simulink model "sltankrule"  (Simulink 4.00)
settings: Solver=ode45  SolverMode=SingleTasking  StartTime=0  StopTime=10000  MaxStep=0.2  RelTol=1e-3  AbsTol=1e-6
PreLoadFcn:
  | tank=readfis('tank');
libraries: fuzblock x1
CloseFcn:
  | AnimFigH = findobj(0,'Name', 'Tank Demo'); close(AnimFigH),ruleFigH = findobj(0,'Name', 'Rule Viewer: tank'); close(ruleFigH)
settings Model: Creator=pascal  LastModifiedBy=eyarrow  SaveTime=off  SaveOutput=off  LimitDataPoints=off  RTWTemplateMakefile=grt_unix.tmf  BlockReductionOpt=off

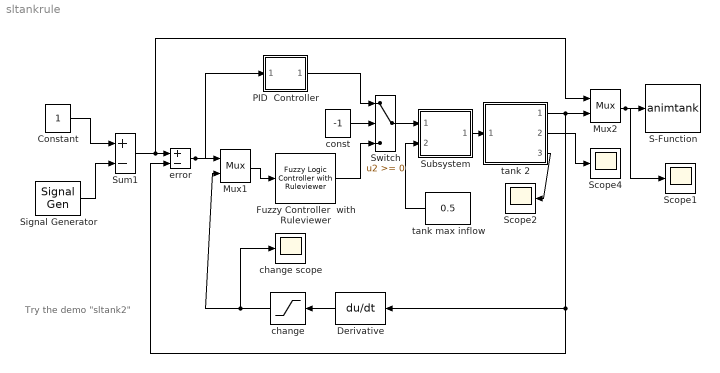
== system sltankrule ==
  note: Try the demo
      | "sltank2"
  Constant : Constant  Value=1
  Derivative : Derivative  Orientation=left
  Fuzzy Controller  with Ruleviewer : fuzblock/Fuzzy Logic  Controller  with Ruleviewer  fismatrix=tank  Ts=2
  Mux1 : Mux  Inputs=2
      settings: DisplayOption=none
  Mux2 : Mux  Inputs=2
      settings: DisplayOption=none
  PID  Controller : Subsystem  mask(PID Controller){@1=2, @2=0, @3=1}
      mask prompts: @1 "Proportional:"; @2 "Integral"; @3 "Derivative:"
      mask help:
      | Enter expressions for proportional, integral, and derivative terms.
      | P+I/s+Ds
      mask init:
      | P=@1; I=@2; D=@3;
      settings: RTWFcnNameOpts=Auto  RTWFileNameOpts=Auto
      mask Help: This block implements a PID controller where parameters are entered for the Proportional, Integral and Derivative terms. Unmask this block to see how it works. The derivative term is implemented using a true derivative block.
      mask Display: disp('PID')
  S-Function : S-Function  FunctionName=animtank  Parameters=1  PortCounts=[]  SFunctionModules=''
  Scope1 : Scope
      settings: TickLabels=on  TimeRange=200.000000  YMin=-2.000000  YMax=2.000000  SaveToWorkspace=off  SaveName=ScopeData  DataFormat=Array  LimitDataPoints=on  MaxDataPoints=5000
  Scope2 : Scope
      settings: TickLabels=on  TimeRange=20.000000  YMin=-2.000000  YMax=2.000000  SaveToWorkspace=off  SaveName=ScopeData  DataFormat=Array  LimitDataPoints=on  MaxDataPoints=5000
  Scope4 : Scope
      settings: TickLabels=on  TimeRange=200.000000  YMin=-2.000000  YMax=2.000000  SaveToWorkspace=off  SaveName=ScopeData  DataFormat=Array  LimitDataPoints=on  MaxDataPoints=5000
  Signal Generator : SignalGenerator  WaveForm=square  Amplitude=0.500000  Frequency=0.100000  Units=rad/sec
  Subsystem : Subsystem  mask(Valve){@1=0}
      mask prompts: @1 "Initial position [0=closed 1=open]:"
      mask help: Valve
      mask init:
      | InitialPosition = @1;
      settings: RTWFcnNameOpts=Auto  RTWFileNameOpts=Auto
      mask Display: disp('VALVE')
  Sum1 : Sum  Inputs=+-  SaturateOnIntegerOverflow=on
  Switch : Switch  Threshold=0
  change : Saturate  Orientation=left  UpperLimit=0.1  LowerLimit=-0.1  LinearizeAsGain=on
  change scope : Scope
      settings: TickLabels=on  TimeRange=20.000000  YMin=-0.100000  YMax=0.100000  SaveToWorkspace=off  SaveName=ScopeData  DataFormat=Array  LimitDataPoints=on  MaxDataPoints=5000
  const : Constant  Value=-1
  error : Sum  Inputs=+-  SaturateOnIntegerOverflow=on
  tank 2 : Subsystem  mask(Water tank){@1=2, @2=1, @3=0.05, @4=0, @5=0.5}
      mask prompts: @1 "Height of tank (m):"; @2 "Bottom area (m^2):"; @3 "Out pipe crossection (m^2):"; @4 "Overflow sensor distance from top (m):"; @5 "Initial level height (m):"
      mask help: Cylindrical water tank with overflow signal
      mask init:
      | ht=@1;area=@2;outletArea=@3;overflowLimit=@4;initialHt=@5;
      settings: RTWFcnNameOpts=Auto  RTWFileNameOpts=Auto
      mask Display: disp('WATER\nTANK')
  tank max inflow : Constant  Orientation=left  Value=0.5
  wires:
  tank 2/2(flow out) -> Scope4/1
  tank max inflow/1 -> Subsystem/2(source flow)
  Derivative/1 -> change/1
  Mux1/1 -> Fuzzy Controller  with Ruleviewer/1
  change/1 -> Mux1/2, change scope/1
  Constant/1 -> Sum1/1
  Signal Generator/1 -> Sum1/2
  Subsystem/1(out flow) -> tank 2/1(flow in)
  tank 2/1(water level) -> Mux2/2, error/2, Derivative/1
  Sum1/1 -> error/1, Mux2/1
  tank 2/3(overflow flag) -> Scope2/1
  Switch/1 -> Subsystem/1(control)
  Mux2/1 -> S-Function/1, Scope1/1
  error/1 -> Mux1/1, PID  Controller/1(In_1)
  Fuzzy Controller  with Ruleviewer/1 -> Switch/3
  PID  Controller/1(Out_1) -> Switch/1
  const/1 -> Switch/2

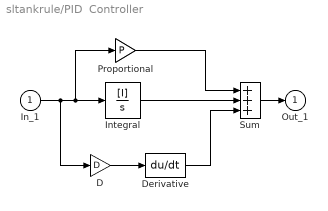
== system sltankrule/PID  Controller ==
  In_1 : Inport  Port=1  LatchInput=off
  D : Gain  Gain=D  Multiplication=Element-wise(K.*u)  SaturateOnIntegerOverflow=on
  Derivative : Derivative
  Integral : TransferFcn  Numerator=[I]  Denominator=[1 0]  AbsoluteTolerance=auto  Realization=auto
  Proportional : Gain  Gain=P  Multiplication=Element-wise(K.*u)  SaturateOnIntegerOverflow=on
  Sum : Sum  Inputs=+++  SaturateOnIntegerOverflow=on
  Out_1 : Outport  Port=1  InitialOutput=0
  wires:
  Proportional/1 -> Sum/1
  Integral/1 -> Sum/2
  Derivative/1 -> Sum/3
  In_1/1 -> Integral/1, Proportional/1, D/1
  Sum/1 -> Out_1/1
  D/1 -> Derivative/1

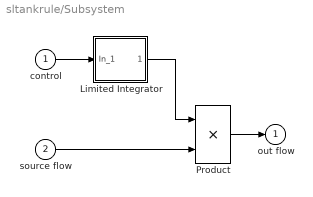
== system sltankrule/Subsystem ==
  control : Inport  Port=1  LatchInput=off
  source flow : Inport  Port=2  LatchInput=off
  Limited Integrator : Subsystem  mask(Limited integrator.){@1=0, @2=1, @3=InitialPosition}
      mask prompts: @1 "Lower bound:"; @2 "Upper bound:"; @3 "Initial condition"
      mask help: Limited integrator
      mask init:
      | lb = @1; ub = @2; xi = @3;
      settings: RTWFcnNameOpts=Auto  RTWFileNameOpts=Auto
      mask Help: Implements a limited integrator with \nan expression of the form:\n\nif(x<=lb and u<0) or (x>=ub and u>0)\n\txdot=0\nelse\n\txdot=u.
      mask Display: plot(-1,-0.2,3.5,1.2,[0.05,1,2,2.9],[0,0,1,1]);disp(' 1/s    ')
  Product : Product  Inputs=2  Multiplication=Element-wise(.*)  SaturateOnIntegerOverflow=on
  out flow : Outport  Port=1  InitialOutput=0
  wires:
  source flow/1 -> Product/2
  Product/1 -> out flow/1
  control/1 -> Limited Integrator/1(In_1)
  Limited Integrator/1(Out_1) -> Product/1

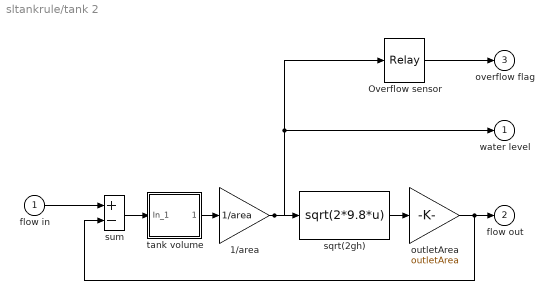
== system sltankrule/tank 2 ==
  flow in : Inport  Port=1  LatchInput=off
  1/area : Gain  Gain=1/area  Multiplication=Element-wise(K.*u)  SaturateOnIntegerOverflow=on
  Overflow sensor : Relay  OnSwitchValue=ht - overflowLimit  OffSwitchValue=ht - overflowLimit  OnOutputValue=1  OffOutputValue=0
  outletArea : Gain  Gain=outletArea  Multiplication=Element-wise(K.*u)  SaturateOnIntegerOverflow=on
  sqrt(2gh) : Fcn  Expr=sqrt(2*9.8*u)
  sum : Sum  Inputs=+-  SaturateOnIntegerOverflow=on
  tank volume : Subsystem  mask(Limited integrator.){@1=0, @2=ht * area, @3=initialHt * area}
      mask prompts: @1 "Lower bound:"; @2 "Upper bound:"; @3 "Initial condition"
      mask help: Limited integrator
      mask init:
      | lb = @1; ub = @2; xi = @3;
      settings: RTWFcnNameOpts=Auto  RTWFileNameOpts=Auto
      mask Help: Implements a limited integrator with \nan expression of the form:\n\nif(x<=lb and u<0) or (x>=ub and u>0)\n\txdot=0\nelse\n\txdot=u.
      mask Display: plot(-1,-0.2,3.5,1.2,[0.05,1,2,2.9],[0,0,1,1]);disp(' 1/s    ')
  water level : Outport  Port=1  InitialOutput=0
  flow out : Outport  Port=2  InitialOutput=0
  overflow flag : Outport  Port=3  InitialOutput=0
  wires:
  outletArea/1 -> flow out/1, sum/2
  sqrt(2gh)/1 -> outletArea/1
  1/area/1 -> Overflow sensor/1, water level/1, sqrt(2gh)/1
  tank volume/1(Out_1) -> 1/area/1
  Overflow sensor/1 -> overflow flag/1
  flow in/1 -> sum/1
  sum/1 -> tank volume/1(In_1)

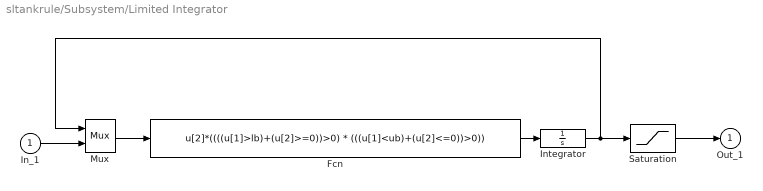
== system sltankrule/Subsystem/Limited Integrator ==
  In_1 : Inport  Port=1  LatchInput=off
  Fcn : Fcn  Expr=u[2]*((((u[1]>lb)+(u[2]>=0))>0) * (((u[1]<ub)+(u[2]<=0))>0))
  Integrator : Integrator  ExternalReset=none  InitialConditionSource=internal  InitialCondition=xi  LimitOutput=off  UpperSaturationLimit=inf  LowerSaturationLimit=-inf  ShowSaturationPort=off  ShowStatePort=off  AbsoluteTolerance=auto
  Mux : Mux  Inputs=2
      settings: DisplayOption=none
  Saturation : Saturate  UpperLimit=ub  LowerLimit=lb  LinearizeAsGain=on
  Out_1 : Outport  Port=1  InitialOutput=0
  wires:
  Integrator/1 -> Saturation/1, Mux/1
  Fcn/1 -> Integrator/1
  Mux/1 -> Fcn/1
  In_1/1 -> Mux/2
  Saturation/1 -> Out_1/1

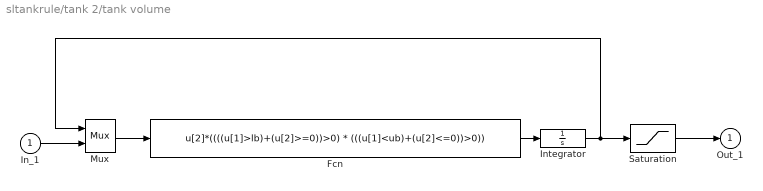
== system sltankrule/tank 2/tank volume ==
  In_1 : Inport  Port=1  LatchInput=off
  Fcn : Fcn  Expr=u[2]*((((u[1]>lb)+(u[2]>=0))>0) * (((u[1]<ub)+(u[2]<=0))>0))
  Integrator : Integrator  ExternalReset=none  InitialConditionSource=internal  InitialCondition=xi  LimitOutput=off  UpperSaturationLimit=inf  LowerSaturationLimit=-inf  ShowSaturationPort=off  ShowStatePort=off  AbsoluteTolerance=auto
  Mux : Mux  Inputs=2
      settings: DisplayOption=none
  Saturation : Saturate  UpperLimit=ub  LowerLimit=lb  LinearizeAsGain=on
  Out_1 : Outport  Port=1  InitialOutput=0
  wires:
  Integrator/1 -> Saturation/1, Mux/1
  Fcn/1 -> Integrator/1
  Mux/1 -> Fcn/1
  In_1/1 -> Mux/2
  Saturation/1 -> Out_1/1
